simulink model "H8_pruebas_SIL"  (R2022b)
settings: Solver=VariableStepAuto  StartTime=0.0  StopTime=5  MaxStep=1e-3  RelTol=1e-3
InitFcn:
  | load("ems.mat");
  | load("hems.mat");
  | load('fuerzasY_LIM.mat')
  | load('matrices_linealizacion_6gdl.mat')
  | m = 200;
  | g = 9.81;
  | 
  | x_lev12 = 0.50086;
  | x_lev34 = 0.48414;
  | x_guid12 = 0.50503;
  | x_guid34 = 0.48831;
  | x_lim = 0.00778;
  | 
  | y_lev13 = 0.23523;
  | y_lev24 = 0.23827;
  | y_guid13 = 0.2372;
  | y_guid24 = 0.2402;
  | y_lim = 0.00154;
  | y_brk = 0.21552;
  | 
  | z_lev = 0.07138;
  | z_guid = 0.04113;
  | z_lim = 0.09146;
  | z_brk = 0.03941;
  | 
  | kp_lev = 50;
  | ki_lev = 400;
  | kp_guid = 6;
  | ki_guid = 46.5;
  | 
  | Imax_lev = 50;
  | Imin_lev = -50;
  | Imax_guid = 50;
  | Imin_guid = 0;
  | 
  | cg_nom=0.61448;
  | lev_nom=0.01965;
  | cg_suelo=0.61733;
  | cg_techo=0.60483;
  | 
  | I = [43.082 0 0; 0 26.887 -0; 0 0 29.297];
  | 
  | fs_current = 20000;
  | fl_current = 10000;
  | var_current = 0.052125100064495;
  | offset_current = 0.001065378087271;
  | 
  | fs_airgap = 20000;
  | fl_airgap = 7500;
  | var_airgap = 1.112140361208638e-08;
  | offset_airgap = 0;
  | airgap_min = 80/1000;
  | airgap_max = 115/1000;
  | 
  | current_filter_order = 20;
  | 
  | airgap_filter_order = 20;
  | N=16;
values from neighbouring files (symbols this model uses):
  A6 = [0 0 0 0 0 0 0 0 0 0 0 0 ... (100 elements, 10x10)]    [matrices_linealizacion_6gdl.mat]    (also in matrices_linealizacion_6gdl2.mat)
  B6 = [0 0 0 0 0 0 -0.0459993641186 -0.0505798680894 0.151580453785 0 0 0 ... (80 elements, 10x8)]    [matrices_linealizacion_6gdl.mat]    (also in matrices_linealizacion_6gdl2.mat)
  C6 = [1 0 0 0 0 0 0 0 0 0 0 1 ... (100 elements, 10x10)]    [matrices_linealizacion_6gdl.mat]    (also in matrices_linealizacion_6gdl2.mat)
  current = [0 10 20 30 40 50 60 70 80 90 100]    [fuerzasY_LIM.mat]
  D6 = [0 0 0 0 0 0 0 0 0 0 0 0 ... (80 elements, 10x8)]    [matrices_linealizacion_6gdl.mat]    (also in matrices_linealizacion_6gdl2.mat)
  FuerzaRail_Y = [0 0 0 0 0 0 0 0.015951701 0.168531476 0.364402347 0.577209778 0.832001165 ... (77 elements, 7x11)]    [fuerzasY_LIM.mat]
  hems =     [hems.mat]
  Ka = [0 0 0 0 4539.83149439 -4539.83149439 4539.83149439 -4539.83149439 -5130.48383819 -5130.48383819 -5130.48383819 -5130.48383819 ... (120 elements, 8x15)]    [Ka_reajustada.mat]    (also in matrices_linealizacion_6gdl.mat = [0 0 0 0 6002.75566687 -6002.75566687 6002.75566687 -6002.75; matrices_linealizacion_6gdl2.mat = [0 0 0 0 1200.55113337 -1200.55113337 1200.55113337 -1200.55)
  Y = [0 1 2 3 4 5 6]    [fuerzasY_LIM.mat]
undefined symbols (not defined in the file or in its folder): DiscIntNeverNeededParam, ems, magnitude
libraries: slpidlib x16, simulink x5
(part 1 of 2)
settings Model: Creator=USUARIO  LastModifiedBy=USUARIO
settings SolverCC: ZeroCrossAlgorithm=Adaptive
settings DebuggingCC: ModelReferenceExtraNoncontSigs=warning

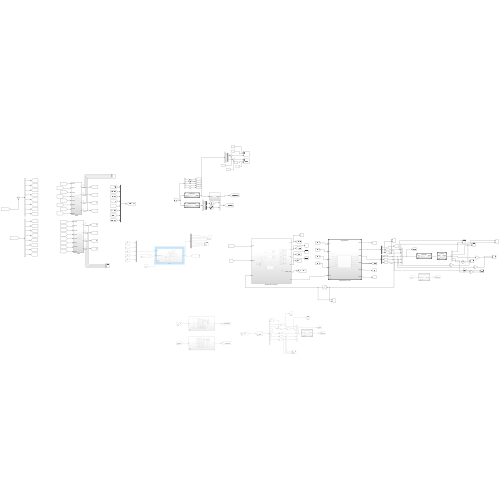
[thumbnail: Simulink's stored preview of the top-level diagram]
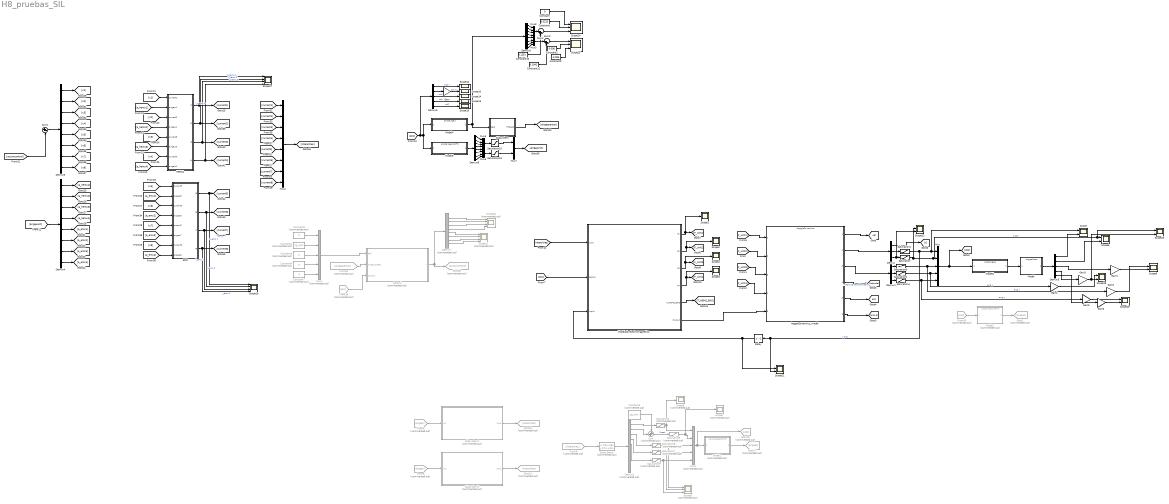
== system H8_pruebas_SIL ==
  Constant : Constant  Value=0
  Constant1 : Constant  Value=0.0225
  Constant10 : Constant  Value=0.1251
  Constant11 : Constant  Value=0.1042
  Constant2 : Constant  Value=0.006
  Constant3 : Constant  Commented=on  Value=cg_nom
  Constant4 : Constant  Commented=on  Value=cg_nom
  Constant{5..8} (4 alike) : Constant  Commented=on  Value=0
  Constant9 : Constant  Value=-0.006
  Control : Subsystem  Commented=on
  Delay : Delay  DelayLength=1  InitialCondition=0.001
  Demux : Demux  Outputs=3
  Demux1 : Demux  Outputs=3
  Demux2 : Demux  Commented=on  Outputs=10
      settings: DisplayOption=none
  Demux3 : Demux  Outputs=5
  Demux{4..5,8..9} (4 alike) : Demux  Outputs=8
  Demux6 : Demux  Outputs=5
  Demux7 : Demux  Commented=on  Outputs=8
  EMS : Subsystem
  From30 : From  Commented=on  GotoTag=airgapsensor
  From39 : From  Commented=on  GotoTag=pos
  From40 : From  Commented=on  GotoTag=pos
  From6 : From  Commented=on  GotoTag=airgaps
  From8 : From  Commented=on  GotoTag=airgaps
  From9 : From  Commented=on  GotoTag=Intensities
  Gain : Gain  Gain=1000
  Gain{1..6} (6 alike) : Gain  Gain=180/pi
  Goto1 : Goto  Commented=on  GotoTag=airgaps
  Goto13 : Goto  Commented=on  GotoTag=Intensities
  Goto16 : Goto  Commented=on  GotoTag=Intensities
  Goto17 : Goto  Commented=on  GotoTag=airgaps
  Goto18 : Goto  Commented=on  GotoTag=pos
  Goto38 : Goto  Commented=on  GotoTag=accioncontrol
  HEMS1 : Subsystem
  Model : ModelReference  ModelNameDialog=airgap2pos.slx  SimulationMode=Normal  ModelReferenceVersion=1.8
  Model1 : ModelReference  Commented=on  ModelNameDialog=pos2airgapUNITS.slx  SimulationMode=Normal  ModelReferenceVersion=1.5
  Model2 : ModelReference  Commented=on  ModelNameDialog=pos2airgapUNITS.slx  SimulationMode=Normal  ModelReferenceVersion=1.5
  Model4 : ModelReference  ModelNameDialog=pos2airgap.slx  SimulationMode=Normal  ModelReferenceVersion=1.7
  Model5 : ModelReference  ModelNameDialog=pos2airgapUNITS.slx  SimulationMode=Normal  ModelReferenceVersion=1.5
  Model6 : ModelReference  ModelNameDialog=pos2airgap.slx  SimulationMode=Normal  ModelReferenceVersion=1.7
  Modelado electromagnetico : Subsystem
  Mux : Mux  Inputs=5
  Mux1 : Mux  Commented=on  Inputs=5
  Mux2 : Mux  Inputs=8
  Mux{3,5..6,8} (4 alike) : Mux
  Mux4 : Mux  Commented=on  Inputs=5
  Mux7 : Mux  Inputs=2
  Saturation : Saturate  UpperLimit=cg_suelo  LowerLimit=cg_techo
  Saturation1 : Saturate  UpperLimit=0.012  LowerLimit=-0.012
  Saturation15 : Saturate  UpperLimit=0.0225  LowerLimit=0.01
  Saturation16 : Saturate  UpperLimit=0.024  LowerLimit=0
  Saturation2 : Saturate  UpperLimit=0.01268  LowerLimit=-0.01268
  Saturation3 : Saturate  UpperLimit=0.0476  LowerLimit=-0.0476
  Saturation4 : Saturate  UpperLimit=0.024  LowerLimit=-0.024
  Saturation5 : Saturate  Commented=on  UpperLimit=cg_suelo  LowerLimit=cg_techo
  Saturation6 : Saturate  Commented=on  UpperLimit=0.012  LowerLimit=-0.012
  Saturation7 : Saturate  Commented=on  UpperLimit=0.01268  LowerLimit=-0.01268
  Saturation8 : Saturate  Commented=on  UpperLimit=0.0476  LowerLimit=-0.0476
  Saturation9 : Saturate  Commented=on  UpperLimit=0.024  LowerLimit=-0.024
  Scope{,5..6,18..19,21..23} (8 alike) : Scope  NumInputPorts=2
  Scope{1..4,10,12..15} (9 alike) : Scope
  Scope11 : Scope  Commented=on  NumInputPorts=4
  Scope16 : Scope  NumInputPorts=4
  Scope24 : Scope  NumInputPorts=3
  Scope25 : Scope  NumInputPorts=3
  Scope26 : Scope  Commented=on  NumInputPorts=4
  Scope27 : Scope  NumInputPorts=4
  Scope7 : Scope  Commented=on
  Scope8 : Scope  Commented=on
  Scope9 : Scope  Commented=on  NumInputPorts=3
  State-Space : StateSpace  Commented=on  A=A6  B=B6  C=C6  D=D6  InitialCondition=[-0.001 0.001 0.001 -0.001 0.001 0 0 0 0 0]
  Subsystem : Subsystem
  Subsystem1 : Subsystem  Commented=on
  Subsystem2 : Subsystem  Commented=on
  Sum : Sum  Commented=on  Inputs=++|
  Sum1 : Sum  Inputs=|+-
  Sum2 : Sum  Inputs=|-+
  Sum3 : Sum  Inputs=|-+
  boggieDynamics_model : ModelReference  ModelNameDialog=boggieDynamics.mdl  SimulationMode=Normal  ModelReferenceVersion=1.43
  tag scope: acc=global, vel=global
  wires:
  [F_Unit4] -> boggieDynamics_model/4
  [F_Unit3] -> boggieDynamics_model/3
  [F_Unit2] -> boggieDynamics_model/2
  boggieDynamics_model/4 -> [Attitude]  "matriz de transformacion"
  [F_Unit1] -> boggieDynamics_model/1
  boggieDynamics_model/3 -> Demux1/1
  Mux/1 -> Model6/1, [pos]
  boggieDynamics_model/2 -> Demux/1
  Demux/3 -> Scope22/2, Saturation/1
  Demux/1 -> [x]
  boggieDynamics_model/1 -> [vel]
  Demux/2 -> Saturation1/1
  boggieDynamics_model/5 -> [acc]
  boggieDynamics_model/6 -> [angvel]
  [pos] -> Modelado electromagnetico/2(Ag_lev)
  [Intensities] -> Modelado electromagnetico/1(I_lev)
  Modelado electromagnetico/3(F3) -> Scope4/1, [F_Unit3]
  Modelado electromagnetico/2(F2) -> Scope2/1, [F_Unit2]
  Modelado electromagnetico/1(F1) -> Scope1/1, [F_Unit1]
  Modelado electromagnetico/5(T_HEMS_EMS) -> [T_HEMS_EMS]
  Demux1/1 -> Saturation3/1
  Demux1/2 -> Saturation2/1
  Demux1/3 -> Saturation4/1
  Model2/1 -> Goto1/1
  Saturation1/1 -> Scope21/2, Delay/1, Scope/1, Mux/1  "y pos"
  Saturation/1 -> Scope22/1, Scope23/1, Scope5/1, Mux/2  "z pos"
  Saturation3/1 -> Gain2/1, Mux/3  "ang x"
  Saturation2/1 -> Gain4/1, Mux/4  "ang y"
  Saturation4/1 -> Gain5/1, Mux/5  "ang z"
  Modelado electromagnetico/4(F4) -> Scope3/1, [F_Unit4]
  Subsystem1/1(Out1) -> Goto16/1
  From8/1 -> Subsystem1/1(In1)
  From6/1 -> Subsystem2/1(In1)
  Subsystem2/1(Out1) -> Goto13/1
  From9/1 -> State-Space/1
  State-Space/1 -> Demux2/1
  Demux2/3 -> Saturation8/1
  Saturation7/1 -> Scope9/2, Mux1/4
  Saturation8/1 -> Mux1/3, Scope9/1
  Demux2/4 -> Saturation7/1
  Saturation9/1 -> Mux1/5, Scope9/3
  Model1/1 -> Goto17/1
  Demux2/5 -> Saturation9/1
  Saturation6/1 -> Mux1/1, Scope8/1
  Demux2/1 -> Saturation6/1
  Mux1/1 -> Model1/1, Goto18/1
  Constant3/1 -> Sum/1
  Demux2/2 -> Sum/2
  Sum/1 -> Saturation5/1  "lineal"
  Saturation5/1 -> Mux1/2, Scope7/1
  Demux4/5 -> [a_ems1]
  [a_hems1] -> HEMS1/2(airgap1)
  Demux4/7 -> [a_ems3]
  [current8] -> Mux2/8
  Demux4/8 -> [a_ems4]
  Demux5/5 -> [c5]
  Demux4/6 -> [a_ems2]
  [accioncontrol] -> Sum1/2
  From30/1 -> Control/2(airgaps_Real)
  Demux4/2 -> [a_hems2]
  Demux5/2 -> [c2]
  Demux5/4 -> [c4]
  Mux7/1 -> [airgapunit]
  Saturation16/1 -> Mux7/2
  Saturation15/1 -> Mux7/1
  Demux7/8 -> Scope11/4
  Mux5/1 -> Saturation16/1
  Demux8/6 -> Mux5/2
  Demux8/7 -> Mux5/3
  Mux6/1 -> Saturation15/1
  Demux8/3 -> Mux6/3
  Demux8/5 -> Mux5/1
  Demux5/3 -> [c3]
  Demux8/2 -> Mux6/2
  Sum1/1 -> Demux5/1
  [current5] -> Mux2/5
  Demux6/3 -> Scope14/1  "rotX"
  [current6] -> Mux2/6
  [current7] -> Mux2/7
  Demux7/5 -> Scope11/1
  Constant5/1 -> Mux4/3
  [a_ems1] -> EMS/2(airgap5)
  Mux4/1 -> Control/1(Ref)
  Demux6/5 -> Scope15/1  "rotZ"
  Demux5/1 -> [c1]
  Demux7/6 -> Scope11/2
  Constant6/1 -> Mux4/4
  [current1] -> Mux2/1
  [a_hems3] -> HEMS1/6(airgap3)
  [a_ems3] -> EMS/6(airgap7)
  [a_hems4] -> HEMS1/8(airgap4)
  Demux4/1 -> [a_hems1]
  [a_ems4] -> EMS/8(airgap8)
  [a_hems2] -> HEMS1/4(airgap2)
  Demux5/7 -> [c7]
  [current3] -> Mux2/3
  Model4/1 -> Demux9/1, Subsystem/1(Real)
  Demux6/4 -> Scope13/1  "rotY"
  Demux7/7 -> Scope11/3
  Demux4/4 -> [a_hems4]
  Gain/1 -> Scope10/1  "pos Z"
  Constant4/1 -> Mux4/2
  Constant8/1 -> Mux4/1
  Demux5/6 -> [c6]
  Constant7/1 -> Mux4/5
  Demux4/3 -> [a_hems3]
  Demux8/8 -> Mux5/4
  Demux6/2 -> Gain/1
  Demux8/1 -> Mux6/1
  [current2] -> Mux2/2
  [a_ems2] -> EMS/4(airgap6)
  [current4] -> Mux2/4
  Demux5/8 -> [c8]
  Mux2/1 -> [Intensities]
  Demux6/1 -> Scope12/1  "pos Y"
  Demux8/4 -> Mux6/4
  [airgapunit] -> Demux4/1
  [pos] -> Demux6/1, Model4/1, Model5/1
  Model5/1 -> Demux8/1
  Control/1(I) -> Goto38/1, Demux7/1
  From39/1 -> Control/3(Output)
  From40/1 -> Model2/1
  Model6/1 -> Model/1
  Model/1 -> Demux3/1
  Demux3/1 -> Scope/2
  Demux3/2 -> Scope5/2
  Demux3/3 -> Gain1/1
  Demux3/4 -> Gain3/1
  Demux3/5 -> Gain6/1
  Modelado electromagnetico/6(Output) -> boggieDynamics_model/5
  Delay/1 -> Scope21/1, Modelado electromagnetico/3(Input)
  Gain1/1 -> Scope6/2
  Gain2/1 -> Scope6/1
  Gain3/1 -> Scope23/2, Scope18/2
  Gain4/1 -> Scope18/1
  Gain5/1 -> Scope19/1
  Gain6/1 -> Scope19/2
  Demux9/6 -> Mux3/2
  Demux9/8 -> Mux3/4
  Demux9/4 -> Mux8/4
  Demux9/7 -> Mux3/3
  Demux9/5 -> Mux3/1
  Demux9/3 -> Mux8/3
  Demux9/1 -> Mux8/1
  Mux3/1 -> Sum3/1
  Mux8/1 -> Sum2/1
  Demux9/2 -> Mux8/2
  Sum2/1 -> Scope24/3
  Constant1/1 -> Scope24/2
  Constant/1 -> Scope24/1
  Sum3/1 -> Scope25/1
  Constant9/1 -> Scope25/3
  Constant2/1 -> Scope25/2
  Constant10/1 -> Sum2/2
  Constant11/1 -> Sum3/2
  Demux7/1 -> Scope26/1
  Demux7/2 -> Scope26/2
  Demux7/3 -> Scope26/3
  Demux7/4 -> Scope26/4
  [c4] -> HEMS1/7(current4)
  [c3] -> HEMS1/5(current3)
  [c2] -> HEMS1/3(current2)
  [c1] -> HEMS1/1(current1)
  HEMS1/1(I1) -> Scope27/1, [current1]  "I_hems 1"
  HEMS1/2(I2) -> Scope27/2, [current2]  "I_hems 2"
  HEMS1/3(I3) -> Scope27/3, [current3]  "I_hems 3"
  HEMS1/4(I4) -> Scope27/4, [current4]  "I_hems 4"
  EMS/1(I5) -> Scope16/1, [current5]  "I_ems 1"
  EMS/2(I6) -> Scope16/2, [current6]  "I_ems 1"
  EMS/3(I7) -> Scope16/3, [current7]  "I_ems 1"
  EMS/4(I8) -> Scope16/4, [current8]  "I_ems 1"
  [c8] -> EMS/7(current8)
  [c7] -> EMS/5(current7)
  [c6] -> EMS/3(current6)
  [c5] -> EMS/1(current5)
  Subsystem/1(Filtered) -> [airgapsensor]

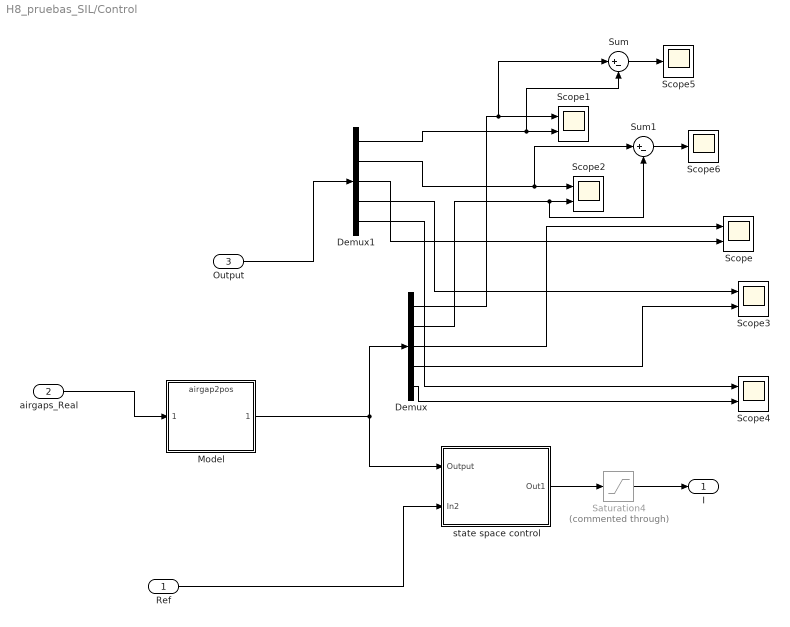
== system H8_pruebas_SIL/Control ==
  Ref : Inport
  airgaps_Real : Inport  Port=2
  Output : Inport  Port=3
  Demux : Demux  Outputs=5
  Demux1 : Demux  Outputs=5
  Model : ModelReference  ModelNameDialog=airgap2pos.slx  SimulationMode=Normal  ModelReferenceVersion=1.8
  Saturation4 : Saturate  Commented=through  UpperLimit=55  LowerLimit=-55
  Scope{,1..4} (5 alike) : Scope  NumInputPorts=2
  Scope5 : Scope
  Scope6 : Scope
  Sum : Sum  Inputs=|+-
  Sum1 : Sum  Inputs=|+-
  state space control : Subsystem
  I : Outport
  wires:
  airgaps_Real/1 -> Model/1
  Saturation4/1 -> I/1
  Model/1 -> state space control/1(Output), Demux/1
  Ref/1 -> state space control/2(In2)
  state space control/1(Out1) -> Saturation4/1
  Demux/1 -> Sum/1, Scope1/1
  Demux/3 -> Scope/1
  Demux/4 -> Scope3/2
  Demux/2 -> Scope2/2, Sum1/2
  Demux1/1 -> Sum/2, Scope1/2
  Demux1/2 -> Sum1/1, Scope2/1
  Demux1/3 -> Scope/2
  Demux1/4 -> Scope3/1
  Demux1/5 -> Scope4/1
  Demux/5 -> Scope4/2
  Sum/1 -> Scope5/1
  Sum1/1 -> Scope6/1
  Output/1 -> Demux1/1

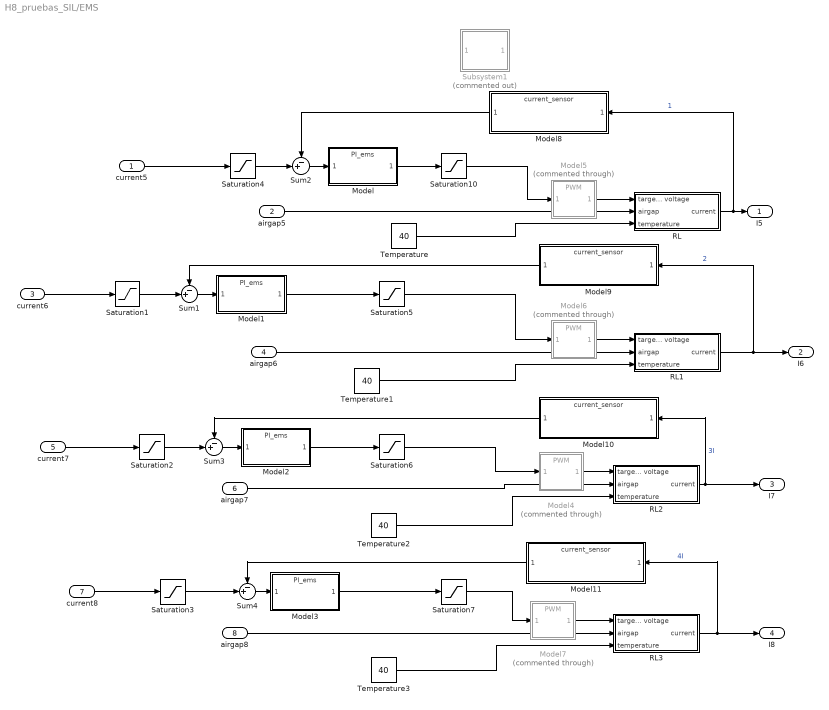
== system H8_pruebas_SIL/EMS ==
  current5 : Inport
  airgap5 : Inport  Port=2
  current6 : Inport  Port=3
  airgap6 : Inport  Port=4
  current7 : Inport  Port=5
  airgap7 : Inport  Port=6
  current8 : Inport  Port=7
  airgap8 : Inport  Port=8
  Model{,1..3} (4 alike) : ModelReference  ModelNameDialog=PI_ems.slx  SimulationMode=Normal  ModelReferenceVersion=1.3
  Model{8..11} (4 alike) : ModelReference  ModelNameDialog=current_sensor.slx  SimulationMode=Normal  ModelReferenceVersion=1.2
  Model{4..7} (4 alike) : ModelReference  Commented=through  ModelNameDialog=PWM.slx  SimulationMode=Normal  ModelReferenceVersion=1.7
  RL : Subsystem
  RL1 : Subsystem
  RL2 : Subsystem
  RL3 : Subsystem
  Saturation{1..4} (4 alike) : Saturate  UpperLimit=50  LowerLimit=0
  Saturation{5..7,10} (4 alike) : Saturate  UpperLimit=200  LowerLimit=-200
  Subsystem1 : Subsystem  Commented=on
  Sum{1..4} (4 alike) : Sum  Inputs=-+|
  Temperature{,1..3} (4 alike) : Constant  Value=40
  I5 : Outport
  I6 : Outport  Port=2
  I7 : Outport  Port=3
  I8 : Outport  Port=4
  wires:
  Temperature/1 -> RL/3(temperature)
  airgap5/1 -> RL/2(airgap)
  Temperature3/1 -> RL3/3(temperature)
  RL/1(current) -> I5/1, Model8/1  "1"
  Temperature1/1 -> RL1/3(temperature)
  Temperature2/1 -> RL2/3(temperature)
  RL3/1(current) -> I8/1, Model11/1  "4I"
  airgap6/1 -> RL1/2(airgap)
  RL1/1(current) -> I6/1, Model9/1  "2"
  RL2/1(current) -> I7/1, Model10/1  "3I"
  airgap7/1 -> RL2/2(airgap)
  airgap8/1 -> RL3/2(airgap)
  Sum2/1 -> Model/1
  Sum1/1 -> Model1/1
  Sum3/1 -> Model2/1
  Sum4/1 -> Model3/1
  Model/1 -> Saturation10/1
  Model3/1 -> Saturation7/1
  Model2/1 -> Saturation6/1
  Model1/1 -> Saturation5/1
  Saturation4/1 -> Sum2/2
  Saturation1/1 -> Sum1/2
  Saturation2/1 -> Sum3/2
  Saturation3/1 -> Sum4/2
  current5/1 -> Saturation4/1
  current6/1 -> Saturation1/1
  current7/1 -> Saturation2/1
  current8/1 -> Saturation3/1
  Saturation7/1 -> Model7/1
  Saturation6/1 -> Model4/1
  Saturation5/1 -> Model6/1
  Saturation10/1 -> Model5/1
  Model6/1 -> RL1/1(target voltage)
  Model4/1 -> RL2/1(target voltage)
  Model5/1 -> RL/1(target voltage)
  Model7/1 -> RL3/1(target voltage)
  Model8/1 -> Sum2/1
  Model9/1 -> Sum1/1
  Model10/1 -> Sum3/1
  Model11/1 -> Sum4/1

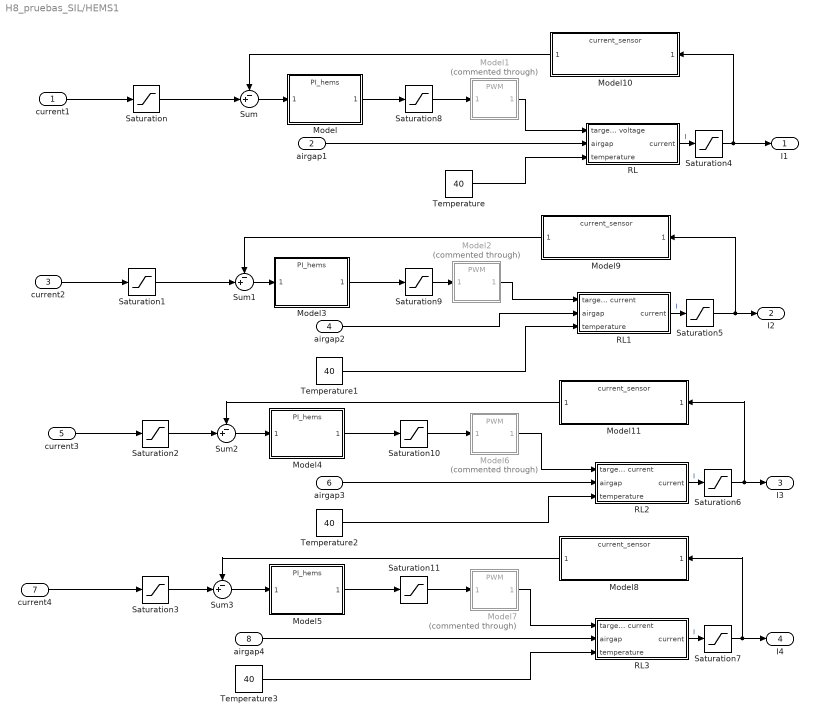
== system H8_pruebas_SIL/HEMS1 ==
  current1 : Inport
  airgap1 : Inport  Port=2
  current2 : Inport  Port=3
  airgap2 : Inport  Port=4
  current3 : Inport  Port=5
  airgap3 : Inport  Port=6
  current4 : Inport  Port=7
  airgap4 : Inport  Port=8
  Model{,3..5} (4 alike) : ModelReference  ModelNameDialog=PI_hems.slx  SimulationMode=Normal  ModelReferenceVersion=1.5
  Model{1..2,6..7} (4 alike) : ModelReference  Commented=through  ModelNameDialog=PWM.slx  SimulationMode=Normal  ModelReferenceVersion=1.7
  Model{8..11} (4 alike) : ModelReference  ModelNameDialog=current_sensor.slx  SimulationMode=Normal  ModelReferenceVersion=1.2
  RL : Subsystem
  RL1 : Subsystem
  RL2 : Subsystem
  RL3 : Subsystem
  Saturation{,1..7} (8 alike) : Saturate  UpperLimit=50  LowerLimit=-50
  Saturation{8..11} (4 alike) : Saturate  UpperLimit=200  LowerLimit=-200
  Sum{,1..3} (4 alike) : Sum  Inputs=-+|
  Temperature{,1..3} (4 alike) : Constant  Value=40
  I1 : Outport
  I2 : Outport  Port=2
  I3 : Outport  Port=3
  I4 : Outport  Port=4
  wires:
  Temperature/1 -> RL/3(temperature)
  Model3/1 -> Saturation9/1
  Model5/1 -> Saturation11/1
  Model/1 -> Saturation8/1
  airgap1/1 -> RL/2(airgap)
  Temperature3/1 -> RL3/3(temperature)
  RL/1(current) -> Saturation4/1  "I"
  Temperature1/1 -> RL1/3(temperature)
  Temperature2/1 -> RL2/3(temperature)
  Model4/1 -> Saturation10/1
  RL3/1(current) -> Saturation7/1  "I"
  airgap2/1 -> RL1/2(airgap)
  RL1/1(current) -> Saturation5/1  "I"
  RL2/1(current) -> Saturation6/1  "I"
  airgap3/1 -> RL2/2(airgap)
  airgap4/1 -> RL3/2(airgap)
  Sum/1 -> Model/1
  Sum1/1 -> Model3/1
  Sum2/1 -> Model4/1
  Sum3/1 -> Model5/1
  Saturation2/1 -> Sum2/2
  Saturation1/1 -> Sum1/2
  Saturation/1 -> Sum/2
  Saturation3/1 -> Sum3/2
  current1/1 -> Saturation/1
  current4/1 -> Saturation3/1
  current3/1 -> Saturation2/1
  current2/1 -> Saturation1/1
  Saturation4/1 -> I1/1, Model10/1
  Saturation5/1 -> I2/1, Model9/1
  Saturation7/1 -> I4/1, Model8/1
  Saturation6/1 -> I3/1, Model11/1
  Saturation8/1 -> Model1/1
  Saturation9/1 -> Model2/1
  Saturation10/1 -> Model6/1
  Saturation11/1 -> Model7/1
  Model1/1 -> RL/1(target voltage)
  Model2/1 -> RL1/1(target current)
  Model6/1 -> RL2/1(target current)
  Model7/1 -> RL3/1(target current)
  Model8/1 -> Sum3/1
  Model9/1 -> Sum1/1
  Model10/1 -> Sum/1
  Model11/1 -> Sum2/1

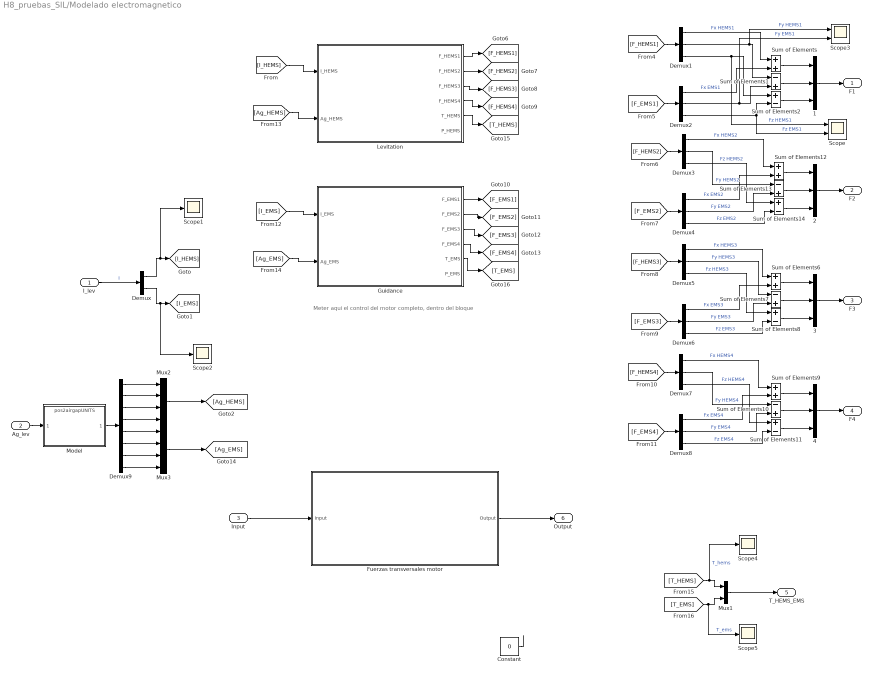
== system H8_pruebas_SIL/Modelado electromagnetico ==
  note: Meter aqui el control del motor completo, dentro del bloque
  I_lev : Inport
  Ag_lev : Inport  Port=2
  Input : Inport  Port=3
  {1..4} (4 alike) : Mux  Inputs=3
  Constant : Constant  Value=0
  Demux : Demux  Outputs=2
  Demux{1..8} (8 alike) : Demux  Outputs=3
  Demux9 : Demux  Outputs=8
  Fuerzas transversales motor : Subsystem
  Guidance : Subsystem
  Levitation : Subsystem
  Model : ModelReference  ModelNameDialog=pos2airgapUNITS.slx  SimulationMode=Normal  ModelReferenceVersion=1.5
  Mux1 : Mux  Inputs=2
  Mux2 : Mux
  Mux3 : Mux
  Scope : Scope  NumInputPorts=2
  Scope{1..2,4..5} (4 alike) : Scope
  Scope3 : Scope  NumInputPorts=2
  Sum of Elements{,6,9,12} (4 alike) : Sum
  Sum of Elements{1,7,10,13} (4 alike) : Sum  Inputs=-+
  Sum of Elements{2,8,11,14} (4 alike) : Sum  Inputs=+-
  F1 : Outport
  F2 : Outport  Port=2
  F3 : Outport  Port=3
  F4 : Outport  Port=4
  T_HEMS_EMS : Outport  Port=5
  Output : Outport  Port=6
  wires:
  I_lev/1 -> Demux/1  "I"
  Demux/1 -> Scope1/1, [I_HEMS]
  Demux/2 -> Scope2/1, [I_EMS]
  [I_HEMS] -> Levitation/1(I_HEMS)
  Levitation/1(F_HEMS1) -> [F_HEMS1]
  Levitation/2(F_HEMS2) -> [F_HEMS2]
  Levitation/3(F_HEMS3) -> [F_HEMS3]
  Levitation/4(F_HEMS4) -> [F_HEMS4]
  Sum of Elements/1 -> 1/1
  1/1 -> F1/1
  Sum of Elements1/1 -> 1/2
  Sum of Elements2/1 -> 1/3
  2/1 -> F2/1
  [F_HEMS1] -> Demux1/1
  Demux1/1 -> Sum of Elements/1  "Fx HEMS1"
  Demux1/2 -> Scope3/1, Sum of Elements1/1  "Fy HEMS1"
  Demux1/3 -> Scope/1, Sum of Elements2/1  "Fz HEMS1"
  3/1 -> F3/1
  Sum of Elements8/1 -> 3/3
  Sum of Elements6/1 -> 3/1
  Sum of Elements7/1 -> 3/2
  4/1 -> F4/1
  Sum of Elements11/1 -> 4/3
  Sum of Elements9/1 -> 4/1
  Sum of Elements10/1 -> 4/2
  Guidance/2(F_EMS2) -> [F_EMS2]
  Guidance/3(F_EMS3) -> [F_EMS3]
  Guidance/4(F_EMS4) -> [F_EMS4]
  Guidance/1(F_EMS1) -> [F_EMS1]
  Demux2/1 -> Sum of Elements/2  "Fx EMS1"
  [F_EMS1] -> Demux2/1
  Demux2/2 -> Scope3/2, Sum of Elements1/2  "Fy EMS1"
  Demux2/3 -> Sum of Elements2/2, Scope/2  "Fz EMS1"
  [F_EMS2] -> Demux4/1
  Demux4/1 -> Sum of Elements12/2  "Fx EMS2"
  Demux4/2 -> Sum of Elements13/2  "Fy EMS2"
  Sum of Elements14/1 -> 2/3
  Demux3/1 -> Sum of Elements12/1  "Fx HEMS2"
  [F_HEMS2] -> Demux3/1
  Demux3/2 -> Sum of Elements13/1  "Fy HEMS2"
  Demux3/3 -> Sum of Elements14/1  "Fz HEMS2"
  Sum of Elements13/1 -> 2/2
  Sum of Elements12/1 -> 2/1
  Demux4/3 -> Sum of Elements14/2  "Fz EMS2"
  Demux5/3 -> Sum of Elements8/1  "Fz HEMS3"
  Demux5/2 -> Sum of Elements7/1  "Fy HEMS3"
  [F_HEMS3] -> Demux5/1
  Demux6/3 -> Sum of Elements8/2  "Fz EMS3"
  [F_EMS3] -> Demux6/1
  Demux6/1 -> Sum of Elements6/2  "Fx EMS3"
  Demux5/1 -> Sum of Elements6/1  "Fx HEMS3"
  Demux6/2 -> Sum of Elements7/2  "Fy EMS3"
  Demux7/3 -> Sum of Elements11/1  "Fz HEMS4"
  Demux8/3 -> Sum of Elements11/2  "Fz EMS4"
  Demux8/2 -> Sum of Elements10/2  "Fy EMS4"
  Demux7/2 -> Sum of Elements10/1  "Fy HEMS4"
  Demux7/1 -> Sum of Elements9/1  "Fx HEMS4"
  Demux8/1 -> Sum of Elements9/2  "Fx EMS4"
  [F_HEMS4] -> Demux7/1
  [F_EMS4] -> Demux8/1
  [I_EMS] -> Guidance/1(I_EMS)
  Ag_lev/1 -> Model/1
  [Ag_HEMS] -> Levitation/2(Ag_HEMS)
  [Ag_EMS] -> Guidance/2(Ag_EMS)
  Levitation/5(T_HEMS) -> [T_HEMS]
  Guidance/5(T_EMS) -> [T_EMS]
  Mux1/1 -> T_HEMS_EMS/1
  [T_HEMS] -> Scope4/1, Mux1/1  "T_hems"
  [T_EMS] -> Scope5/1, Mux1/2  "T_ems"
  Model/1 -> Demux9/1
  Demux9/1 -> Mux2/1
  Demux9/2 -> Mux2/2
  Demux9/3 -> Mux2/3
  Demux9/4 -> Mux2/4
  Mux2/1 -> [Ag_HEMS]
  Demux9/5 -> Mux3/1
  Demux9/7 -> Mux3/3
  Mux3/1 -> [Ag_EMS]
  Demux9/6 -> Mux3/2
  Demux9/8 -> Mux3/4
  Input/1 -> Fuerzas transversales motor/1(Input)
  Fuerzas transversales motor/1(Output) -> Output/1
  Constant/1 -> ?

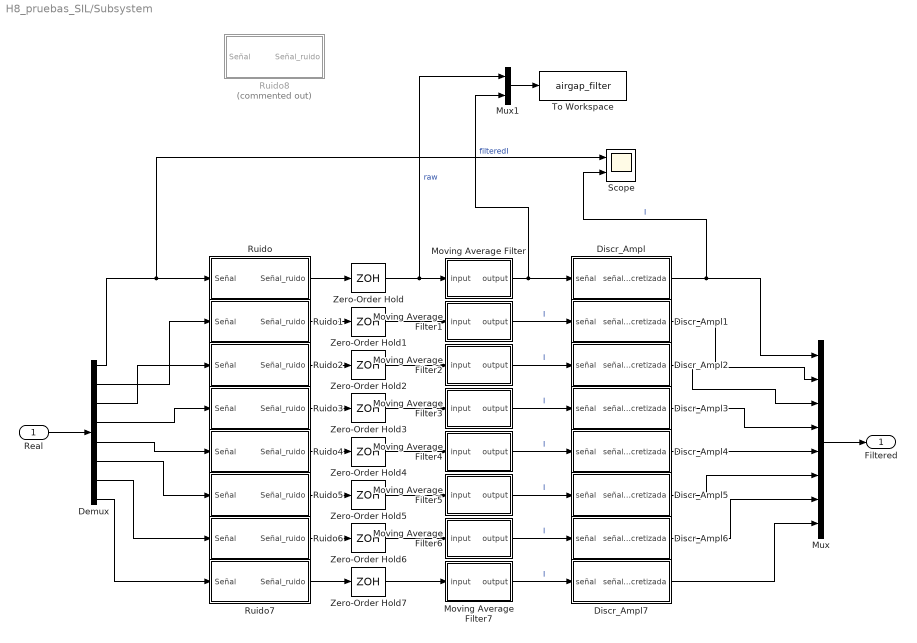
== system H8_pruebas_SIL/Subsystem ==
  Real : Inport
  Demux : Demux  Outputs=8
  Discr_Ampl : Subsystem  mask{N=(2^N)-1, Min=0.045, Max=0.125}
      mask prompts: N "Valores distintos (N)"; Min "Valor mínimo"; Max "Valor máximo"
      mask DialogControl DescGroupVar Prompt: Discretizacion_Amplitud
      mask DialogControl DescTextVar Prompt: Discretización en amplitud
  Discr_Ampl1 : Subsystem  mask{N=(2^N)-1, Min=0.045, Max=0.125}
      mask prompts: N "Valores distintos (N)"; Min "Valor mínimo"; Max "Valor máximo"
      mask DialogControl DescGroupVar Prompt: Discretizacion_Amplitud
      mask DialogControl DescTextVar Prompt: Discretización en amplitud
  Discr_Ampl2 : Subsystem  mask{N=(2^N)-1, Min=0.045, Max=0.125}
      mask prompts: N "Valores distintos (N)"; Min "Valor mínimo"; Max "Valor máximo"
      mask DialogControl DescGroupVar Prompt: Discretizacion_Amplitud
      mask DialogControl DescTextVar Prompt: Discretización en amplitud
  Discr_Ampl3 : Subsystem  mask{N=(2^N)-1, Min=0.045, Max=0.125}
      mask prompts: N "Valores distintos (N)"; Min "Valor mínimo"; Max "Valor máximo"
      mask DialogControl DescGroupVar Prompt: Discretizacion_Amplitud
      mask DialogControl DescTextVar Prompt: Discretización en amplitud
  Discr_Ampl4 : Subsystem  mask{N=(2^N)-1, Min=0.045, Max=0.125}
      mask prompts: N "Valores distintos (N)"; Min "Valor mínimo"; Max "Valor máximo"
      mask DialogControl DescGroupVar Prompt: Discretizacion_Amplitud
      mask DialogControl DescTextVar Prompt: Discretización en amplitud
  Discr_Ampl5 : Subsystem  mask{N=(2^N)-1, Min=0.045, Max=0.125}
      mask prompts: N "Valores distintos (N)"; Min "Valor mínimo"; Max "Valor máximo"
      mask DialogControl DescGroupVar Prompt: Discretizacion_Amplitud
      mask DialogControl DescTextVar Prompt: Discretización en amplitud
  Discr_Ampl6 : Subsystem  mask{N=(2^N)-1, Min=0.045, Max=0.125}
      mask prompts: N "Valores distintos (N)"; Min "Valor mínimo"; Max "Valor máximo"
      mask DialogControl DescGroupVar Prompt: Discretizacion_Amplitud
      mask DialogControl DescTextVar Prompt: Discretización en amplitud
  Discr_Ampl7 : Subsystem  mask{N=(2^N)-1, Min=0.045, Max=0.125}
      mask prompts: N "Valores distintos (N)"; Min "Valor mínimo"; Max "Valor máximo"
      mask DialogControl DescGroupVar Prompt: Discretizacion_Amplitud
      mask DialogControl DescTextVar Prompt: Discretización en amplitud
  Moving Average Filter : Subsystem  mask{M=airgap_filter_order, fs=-1}
      mask prompts: M "Orden del filtro (M)"; fs "Frecuencia de muestreo (fs)"
  Moving Average Filter1 : Subsystem  mask{M=airgap_filter_order, fs=-1}
      mask prompts: M "Orden del filtro (M)"; fs "Frecuencia de muestreo (fs)"
  Moving Average Filter2 : Subsystem  mask{M=airgap_filter_order, fs=-1}
      mask prompts: M "Orden del filtro (M)"; fs "Frecuencia de muestreo (fs)"
  Moving Average Filter3 : Subsystem  mask{M=airgap_filter_order, fs=-1}
      mask prompts: M "Orden del filtro (M)"; fs "Frecuencia de muestreo (fs)"
  Moving Average Filter4 : Subsystem  mask{M=airgap_filter_order, fs=-1}
      mask prompts: M "Orden del filtro (M)"; fs "Frecuencia de muestreo (fs)"
  Moving Average Filter5 : Subsystem  mask{M=airgap_filter_order, fs=-1}
      mask prompts: M "Orden del filtro (M)"; fs "Frecuencia de muestreo (fs)"
  Moving Average Filter6 : Subsystem  mask{M=airgap_filter_order, fs=-1}
      mask prompts: M "Orden del filtro (M)"; fs "Frecuencia de muestreo (fs)"
  Moving Average Filter7 : Subsystem  mask{M=airgap_filter_order, fs=-1}
      mask prompts: M "Orden del filtro (M)"; fs "Frecuencia de muestreo (fs)"
  Mux : Mux  Inputs=8
  Mux1 : Mux  Inputs=2
  Ruido : Subsystem  mask{M=0, V=var_airgap, T=1/fs_airgap}
      mask prompts: M "Media"; V "Varianza"; T "Periodo"
      mask DialogControl Ruido Prompt: Ruido
      mask DialogControl DescTextVar Prompt: Añade ruido gaussiano
  Ruido1 : Subsystem  mask{M=0, V=var_airgap, T=1/fs_airgap}
      mask prompts: M "Media"; V "Varianza"; T "Periodo"
      mask DialogControl Ruido Prompt: Ruido
      mask DialogControl DescTextVar Prompt: Añade ruido gaussiano
  Ruido2 : Subsystem  mask{M=0, V=var_airgap, T=1/fs_airgap}
      mask prompts: M "Media"; V "Varianza"; T "Periodo"
      mask DialogControl Ruido Prompt: Ruido
      mask DialogControl DescTextVar Prompt: Añade ruido gaussiano
  Ruido3 : Subsystem  mask{M=0, V=var_airgap, T=1/fs_airgap}
      mask prompts: M "Media"; V "Varianza"; T "Periodo"
      mask DialogControl Ruido Prompt: Ruido
      mask DialogControl DescTextVar Prompt: Añade ruido gaussiano
  Ruido4 : Subsystem  mask{M=0, V=var_airgap, T=1/fs_airgap}
      mask prompts: M "Media"; V "Varianza"; T "Periodo"
      mask DialogControl Ruido Prompt: Ruido
      mask DialogControl DescTextVar Prompt: Añade ruido gaussiano
  Ruido5 : Subsystem  mask{M=0, V=var_airgap, T=1/fs_airgap}
      mask prompts: M "Media"; V "Varianza"; T "Periodo"
      mask DialogControl Ruido Prompt: Ruido
      mask DialogControl DescTextVar Prompt: Añade ruido gaussiano
  Ruido6 : Subsystem  mask{M=0, V=var_airgap, T=1/fs_airgap}
      mask prompts: M "Media"; V "Varianza"; T "Periodo"
      mask DialogControl Ruido Prompt: Ruido
      mask DialogControl DescTextVar Prompt: Añade ruido gaussiano
  Ruido7 : Subsystem  mask{M=0, V=var_airgap, T=1/fs_airgap}
      mask prompts: M "Media"; V "Varianza"; T "Periodo"
      mask DialogControl Ruido Prompt: Ruido
      mask DialogControl DescTextVar Prompt: Añade ruido gaussiano
  Ruido8 : Subsystem  Commented=on  mask{M=0, V=5e-8, T=0.00001}
      mask prompts: M "Media"; V "Varianza"; T "Periodo"
      mask DialogControl Ruido Prompt: Ruido
      mask DialogControl DescTextVar Prompt: Añade ruido gaussiano
  Scope : Scope  NumInputPorts=2
  To Workspace : ToWorkspace  VariableName=airgap_filter  SaveFormat=Timeseries  SampleTime=-1
  Zero-Order Hold{,1..7} (8 alike) : ZeroOrderHold  SampleTime=1/fl_airgap
  Filtered : Outport
  wires:
  Real/1 -> Demux/1
  Demux/2 -> Ruido1/1(Señal)
  Demux/3 -> Ruido2/1(Señal)
  Demux/4 -> Ruido3/1(Señal)
  Demux/5 -> Ruido4/1(Señal)
  Demux/6 -> Ruido5/1(Señal)
  Demux/7 -> Ruido6/1(Señal)
  Demux/8 -> Ruido7/1(Señal)
  Mux/1 -> Filtered/1
  Discr_Ampl1/1(señal_discretizada) -> Mux/2
  Discr_Ampl2/1(señal_discretizada) -> Mux/3
  Discr_Ampl3/1(señal_discretizada) -> Mux/4
  Discr_Ampl4/1(señal_discretizada) -> Mux/5
  Discr_Ampl5/1(señal_discretizada) -> Mux/6
  Discr_Ampl6/1(señal_discretizada) -> Mux/7
  Discr_Ampl7/1(señal_discretizada) -> Mux/8
  Discr_Ampl/1(señal_discretizada) -> Scope/2, Mux/1  "I"
  Zero-Order Hold/1 -> Mux1/1, Moving Average Filter/1(input)  "raw"
  Ruido/1(Señal_ruido) -> Zero-Order Hold/1
  Moving Average Filter/1(output) -> Mux1/2, Discr_Ampl/1(señal)  "filteredI"
  Ruido1/1(Señal_ruido) -> Zero-Order Hold1/1
  Zero-Order Hold1/1 -> Moving Average Filter1/1(input)
  Moving Average Filter1/1(output) -> Discr_Ampl1/1(señal)  "I"
  Ruido2/1(Señal_ruido) -> Zero-Order Hold2/1
  Zero-Order Hold2/1 -> Moving Average Filter2/1(input)
  Moving Average Filter2/1(output) -> Discr_Ampl2/1(señal)  "I"
  Ruido3/1(Señal_ruido) -> Zero-Order Hold3/1
  Zero-Order Hold3/1 -> Moving Average Filter3/1(input)
  Moving Average Filter3/1(output) -> Discr_Ampl3/1(señal)  "I"
  Ruido4/1(Señal_ruido) -> Zero-Order Hold4/1
  Zero-Order Hold4/1 -> Moving Average Filter4/1(input)
  Moving Average Filter4/1(output) -> Discr_Ampl4/1(señal)  "I"
  Ruido5/1(Señal_ruido) -> Zero-Order Hold5/1
  Zero-Order Hold5/1 -> Moving Average Filter5/1(input)
  Moving Average Filter5/1(output) -> Discr_Ampl5/1(señal)  "I"
  Ruido6/1(Señal_ruido) -> Zero-Order Hold6/1
  Zero-Order Hold6/1 -> Moving Average Filter6/1(input)
  Moving Average Filter6/1(output) -> Discr_Ampl6/1(señal)  "I"
  Ruido7/1(Señal_ruido) -> Zero-Order Hold7/1
  Zero-Order Hold7/1 -> Moving Average Filter7/1(input)
  Moving Average Filter7/1(output) -> Discr_Ampl7/1(señal)  "I"
  Demux/1 -> Ruido/1(Señal), Scope/1
  Mux1/1 -> To Workspace/1

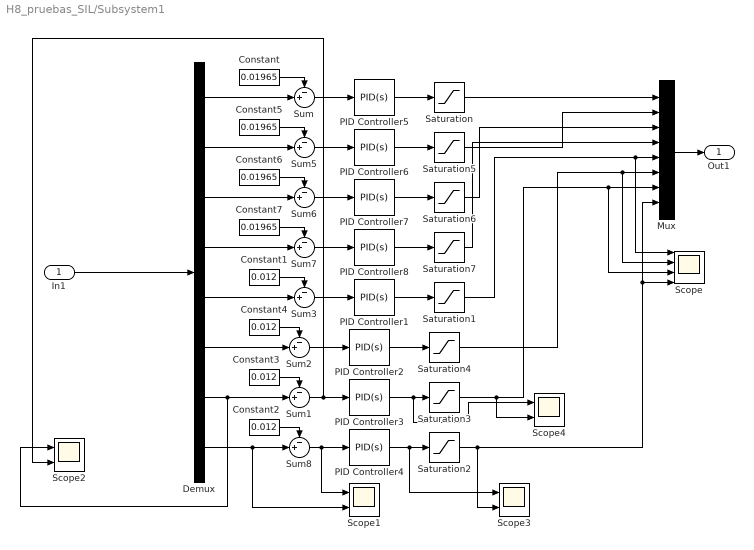
== system H8_pruebas_SIL/Subsystem1 ==
  In1 : Inport
  Constant{,5..7} (4 alike) : Constant  Value=0.01965
  Constant{1..4} (4 alike) : Constant  Value=0.012
  Demux : Demux  Outputs=8
  Mux : Mux  Inputs=8
  PID Controller{1..4} (4 alike) : slpidlib/PID Controller  Controller=PID  Form=Parallel  TimeDomain=Continuous-time  UseExternalTs=off  SampleTime=-1  IntegratorMethod=Forward Euler  FilterMethod=Forward Euler  ControllerParametersSource=internal  P=6490  I=15500  UseKiTs=off  D=100  N=1900  UseFilter=on  TunerSelectOption=Transfer Function Based (PID Tuner App)  InitialConditionSource=internal  InitialConditionForIntegrator=suelo  InitialConditionForFilter=0  DifferentiatorICPrevScaledInput=0  ExternalReset=none  TrackingMode=off  Kt=1  LimitOutput=off  SatLimitsSource=internal  UpperSaturationLimit=inf  LowerSaturationLimit=-inf  LinearizeAsGain=on  AntiWindupMode=none  Kb=1  LimitIntegrator=off  UpperIntegratorSaturationLimit=inf  LowerIntegratorSaturationLimit=-inf  POutMin=[]  POutMax=[]  IOutMin=[]  IOutMax=[]  DOutMin=[]  DOutMax=[]  NOutMin=[]  NOutMax=[]  SumOutMin=[]  SumOutMax=[]  SaturationOutMin=[]  SaturationOutMax=[]  PParamMin=[]  PParamMax=[]  IParamMin=[]  IParamMax=[]  DParamMin=[]  DParamMax=[]  NParamMin=[]  NParamMax=[]  KbParamMin=[]  KbParamMax=[]  KtParamMin=[]  KtParamMax=[]  KbOutMin=[]  KbOutMax=[]  KtOutMin=[]  KtOutMax=[]  IntegratorOutMin=[]  IntegratorOutMax=[]  FilterOutMin=[]  FilterOutMax=[]  SumI1OutMin=[]  SumI1OutMax=[]  SumI2OutMin=[]  SumI2OutMax=[]  SumI3OutMin=[]  SumI3OutMax=[]  SumI4OutMin=[]  SumI4OutMax=[]  SumDOutMin=[]  SumDOutMax=[]  DifferentiatorOutMin=[]  DifferentiatorOutMax=[]  FilterDiffOutCoefMin=[]  FilterDiffOutCoefMax=[]  ReciprocalOutMin=[]  ReciprocalOutMax=[]  SumDenOutMin=[]  SumDenOutMax=[]  SumNumOutMin=[]  SumNumOutMax=[]  DivideOutMin=[]  DivideOutMax=[]  UdiffTsProdOutMin=[]  UdiffTsProdOutMax=[]  NTsProdOutMin=[]  NTsProdOutMax=[]  UintegralTsProdOutMin=[]  UintegralTsProdOutMax=[]  UngainTsProdOutMin=[]  UngainTsProdOutMax=[]  ClampingZeroOutDataTypeStr=Inherit: Inherit via back propagation  ClampingZeroOutMin=[]  ClampingZeroOutMax=[]  FilterDenConstantOutDataTypeStr=Inherit: Inherit via back propagation  FilterDenConstantOutMin=[]  FilterDenConstantOutMax=[]  PCopyOutDataTypeStr=Inherit: Inherit via back propagation  PCopyOutMin=[]  PCopyOutMax=[]  NCopyOutDataTypeStr=Inherit: Inherit via back propagation  NCopyOutMin=[]  NCopyOutMax=[]  IntegratorContinuousStateAttributes=''  IntegratorStateMustResolveToSignalObject=off  IntegratorRTWStateStorageClass=Auto  FilterContinuousStateAttributes=''  FilterStateMustResolveToSignalObject=off  FilterRTWStateStorageClass=Auto  ParallelPVariant=InternalParameters  IdealPVariant=Disabled  IVariant=InternalParameters  DVariant=InternalParameters  IntegratorVariant=Continuous  SatVariant=Disabled  AWVariant=Passthrough  PCopyVariant=Disabled  TRVariant=Disabled  FdbkBlocksVariant=Forward  IdealPFdbkVariant=Disabled  SatFdbkVariant=Disabled  DerivativeFilterVariant=ContFilter  NVariant=InternalParameters  NCopyVariant=Disabled  FilterICVariant=InternalICsFilter  IntegratorICVariant=InternalICs  ExternalResetVariant=Disabled  TRSumVariant=Passthrough  SumFdbkVariant=Disabled  SumVariant=Sum_PID  TsampFilterVariant=InternalTs  TsampNgainVariant=Passthrough  TsampIntegralVariant=Passthrough  ExternalSaturationOutDataTypeStr=Inherit: Same as second input
  PID Controller{5..8} (4 alike) : slpidlib/PID Controller  Controller=PID  Form=Parallel  TimeDomain=Continuous-time  UseExternalTs=off  SampleTime=-1  IntegratorMethod=Forward Euler  FilterMethod=Forward Euler  ControllerParametersSource=internal  P=64900  I=155000  UseKiTs=off  D=1000  N=1900  UseFilter=on  TunerSelectOption=Transfer Function Based (PID Tuner App)  InitialConditionSource=internal  InitialConditionForIntegrator=suelo  InitialConditionForFilter=0  DifferentiatorICPrevScaledInput=0  ExternalReset=none  TrackingMode=off  Kt=1  LimitOutput=off  SatLimitsSource=internal  UpperSaturationLimit=inf  LowerSaturationLimit=-inf  LinearizeAsGain=on  AntiWindupMode=none  Kb=1  LimitIntegrator=off  UpperIntegratorSaturationLimit=inf  LowerIntegratorSaturationLimit=-inf  POutMin=[]  POutMax=[]  IOutMin=[]  IOutMax=[]  DOutMin=[]  DOutMax=[]  NOutMin=[]  NOutMax=[]  SumOutMin=[]  SumOutMax=[]  SaturationOutMin=[]  SaturationOutMax=[]  PParamMin=[]  PParamMax=[]  IParamMin=[]  IParamMax=[]  DParamMin=[]  DParamMax=[]  NParamMin=[]  NParamMax=[]  KbParamMin=[]  KbParamMax=[]  KtParamMin=[]  KtParamMax=[]  KbOutMin=[]  KbOutMax=[]  KtOutMin=[]  KtOutMax=[]  IntegratorOutMin=[]  IntegratorOutMax=[]  FilterOutMin=[]  FilterOutMax=[]  SumI1OutMin=[]  SumI1OutMax=[]  SumI2OutMin=[]  SumI2OutMax=[]  SumI3OutMin=[]  SumI3OutMax=[]  SumI4OutMin=[]  SumI4OutMax=[]  SumDOutMin=[]  SumDOutMax=[]  DifferentiatorOutMin=[]  DifferentiatorOutMax=[]  FilterDiffOutCoefMin=[]  FilterDiffOutCoefMax=[]  ReciprocalOutMin=[]  ReciprocalOutMax=[]  SumDenOutMin=[]  SumDenOutMax=[]  SumNumOutMin=[]  SumNumOutMax=[]  DivideOutMin=[]  DivideOutMax=[]  UdiffTsProdOutMin=[]  UdiffTsProdOutMax=[]  NTsProdOutMin=[]  NTsProdOutMax=[]  UintegralTsProdOutMin=[]  UintegralTsProdOutMax=[]  UngainTsProdOutMin=[]  UngainTsProdOutMax=[]  ClampingZeroOutDataTypeStr=Inherit: Inherit via back propagation  ClampingZeroOutMin=[]  ClampingZeroOutMax=[]  FilterDenConstantOutDataTypeStr=Inherit: Inherit via back propagation  FilterDenConstantOutMin=[]  FilterDenConstantOutMax=[]  PCopyOutDataTypeStr=Inherit: Inherit via back propagation  PCopyOutMin=[]  PCopyOutMax=[]  NCopyOutDataTypeStr=Inherit: Inherit via back propagation  NCopyOutMin=[]  NCopyOutMax=[]  IntegratorContinuousStateAttributes=''  IntegratorStateMustResolveToSignalObject=off  IntegratorRTWStateStorageClass=Auto  FilterContinuousStateAttributes=''  FilterStateMustResolveToSignalObject=off  FilterRTWStateStorageClass=Auto  ParallelPVariant=InternalParameters  IdealPVariant=Disabled  IVariant=InternalParameters  DVariant=InternalParameters  IntegratorVariant=Continuous  SatVariant=Disabled  AWVariant=Passthrough  PCopyVariant=Disabled  TRVariant=Disabled  FdbkBlocksVariant=Forward  IdealPFdbkVariant=Disabled  SatFdbkVariant=Disabled  DerivativeFilterVariant=ContFilter  NVariant=InternalParameters  NCopyVariant=Disabled  FilterICVariant=InternalICsFilter  IntegratorICVariant=InternalICs  ExternalResetVariant=Disabled  TRSumVariant=Passthrough  SumFdbkVariant=Disabled  SumVariant=Sum_PID  TsampFilterVariant=InternalTs  TsampNgainVariant=Passthrough  TsampIntegralVariant=Passthrough  ExternalSaturationOutDataTypeStr=Inherit: Same as second input
  Saturation{,5..7} (4 alike) : Saturate  UpperLimit=50  LowerLimit=-50
  Saturation{1..4} (4 alike) : Saturate  UpperLimit=50  LowerLimit=0
  Scope : Scope  NumInputPorts=4
  Scope{1..4} (4 alike) : Scope  NumInputPorts=2
  Sum{,1..3,5..8} (8 alike) : Sum  Inputs=-+|
  Out1 : Outport
  wires:
  In1/1 -> Demux/1
  Demux/1 -> Sum/2
  Sum/1 -> PID Controller5/1
  Constant/1 -> Sum/1
  PID Controller5/1 -> Saturation/1
  Mux/1 -> Out1/1
  Saturation/1 -> Mux/1
  Saturation1/1 -> Scope/1, Mux/5
  Sum3/1 -> PID Controller1/1
  PID Controller1/1 -> Saturation1/1
  Demux/5 -> Sum3/2
  Constant1/1 -> Sum3/1
  Demux/8 -> Sum8/2, Scope1/2
  PID Controller4/1 -> Scope3/1, Saturation2/1
  Saturation2/1 -> Scope3/2, Scope/4, Mux/8
  Constant2/1 -> Sum8/1
  Demux/7 -> Sum1/2, Scope2/1
  Constant3/1 -> Sum1/1
  PID Controller3/1 -> Scope4/1, Saturation3/1
  Saturation3/1 -> Scope4/2, Scope/3, Mux/7
  Sum1/1 -> PID Controller3/1, Scope2/2
  Demux/6 -> Sum2/2
  Constant4/1 -> Sum2/1
  PID Controller2/1 -> Saturation4/1
  Saturation4/1 -> Scope/2, Mux/6
  Sum2/1 -> PID Controller2/1
  PID Controller6/1 -> Saturation5/1
  Constant5/1 -> Sum5/1
  Demux/2 -> Sum5/2
  Sum5/1 -> PID Controller6/1
  PID Controller7/1 -> Saturation6/1
  Constant6/1 -> Sum6/1
  Saturation6/1 -> Mux/3
  Demux/3 -> Sum6/2
  Sum6/1 -> PID Controller7/1
  Sum7/1 -> PID Controller8/1
  PID Controller8/1 -> Saturation7/1
  Demux/4 -> Sum7/2
  Constant7/1 -> Sum7/1
  Saturation7/1 -> Mux/4
  Saturation5/1 -> Mux/2
  Sum8/1 -> PID Controller4/1, Scope1/1

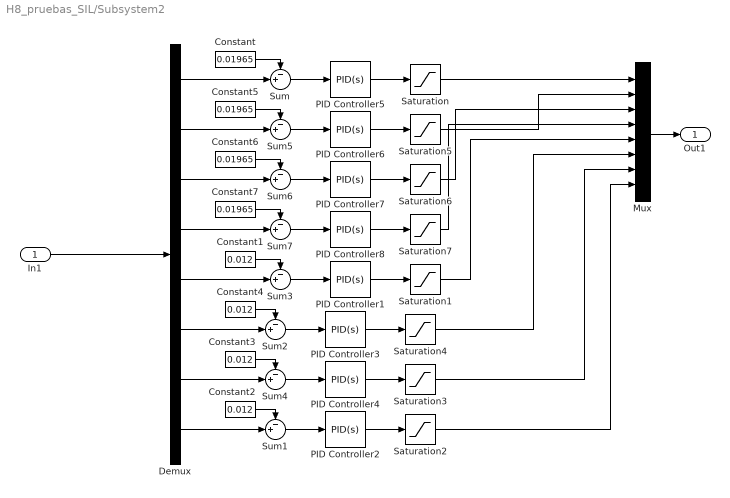
== system H8_pruebas_SIL/Subsystem2 ==
  In1 : Inport
  Constant{,5..7} (4 alike) : Constant  Value=0.01965
  Constant{1..4} (4 alike) : Constant  Value=0.012
  Demux : Demux  Outputs=8
  Mux : Mux  Inputs=8
  PID Controller{1..4} (4 alike) : slpidlib/PID Controller  Controller=PID  Form=Parallel  TimeDomain=Continuous-time  UseExternalTs=off  SampleTime=-1  IntegratorMethod=Forward Euler  FilterMethod=Forward Euler  ControllerParametersSource=internal  P=5490  I=10500  UseKiTs=off  D=350  N=1900  UseFilter=on  TunerSelectOption=Transfer Function Based (PID Tuner App)  InitialConditionSource=internal  InitialConditionForIntegrator=suelo  InitialConditionForFilter=0  DifferentiatorICPrevScaledInput=0  ExternalReset=none  TrackingMode=off  Kt=1  LimitOutput=off  SatLimitsSource=internal  UpperSaturationLimit=inf  LowerSaturationLimit=-inf  LinearizeAsGain=on  AntiWindupMode=none  Kb=1  LimitIntegrator=off  UpperIntegratorSaturationLimit=inf  LowerIntegratorSaturationLimit=-inf  POutMin=[]  POutMax=[]  IOutMin=[]  IOutMax=[]  DOutMin=[]  DOutMax=[]  NOutMin=[]  NOutMax=[]  SumOutMin=[]  SumOutMax=[]  SaturationOutMin=[]  SaturationOutMax=[]  PParamMin=[]  PParamMax=[]  IParamMin=[]  IParamMax=[]  DParamMin=[]  DParamMax=[]  NParamMin=[]  NParamMax=[]  KbParamMin=[]  KbParamMax=[]  KtParamMin=[]  KtParamMax=[]  KbOutMin=[]  KbOutMax=[]  KtOutMin=[]  KtOutMax=[]  IntegratorOutMin=[]  IntegratorOutMax=[]  FilterOutMin=[]  FilterOutMax=[]  SumI1OutMin=[]  SumI1OutMax=[]  SumI2OutMin=[]  SumI2OutMax=[]  SumI3OutMin=[]  SumI3OutMax=[]  SumI4OutMin=[]  SumI4OutMax=[]  SumDOutMin=[]  SumDOutMax=[]  DifferentiatorOutMin=[]  DifferentiatorOutMax=[]  FilterDiffOutCoefMin=[]  FilterDiffOutCoefMax=[]  ReciprocalOutMin=[]  ReciprocalOutMax=[]  SumDenOutMin=[]  SumDenOutMax=[]  SumNumOutMin=[]  SumNumOutMax=[]  DivideOutMin=[]  DivideOutMax=[]  UdiffTsProdOutMin=[]  UdiffTsProdOutMax=[]  NTsProdOutMin=[]  NTsProdOutMax=[]  UintegralTsProdOutMin=[]  UintegralTsProdOutMax=[]  UngainTsProdOutMin=[]  UngainTsProdOutMax=[]  ClampingZeroOutDataTypeStr=Inherit: Inherit via back propagation  ClampingZeroOutMin=[]  ClampingZeroOutMax=[]  FilterDenConstantOutDataTypeStr=Inherit: Inherit via back propagation  FilterDenConstantOutMin=[]  FilterDenConstantOutMax=[]  PCopyOutDataTypeStr=Inherit: Inherit via back propagation  PCopyOutMin=[]  PCopyOutMax=[]  NCopyOutDataTypeStr=Inherit: Inherit via back propagation  NCopyOutMin=[]  NCopyOutMax=[]  IntegratorContinuousStateAttributes=''  IntegratorStateMustResolveToSignalObject=off  IntegratorRTWStateStorageClass=Auto  FilterContinuousStateAttributes=''  FilterStateMustResolveToSignalObject=off  FilterRTWStateStorageClass=Auto  ParallelPVariant=InternalParameters  IdealPVariant=Disabled  IVariant=InternalParameters  DVariant=InternalParameters  IntegratorVariant=Continuous  SatVariant=Disabled  AWVariant=Passthrough  PCopyVariant=Disabled  TRVariant=Disabled  FdbkBlocksVariant=Forward  IdealPFdbkVariant=Disabled  SatFdbkVariant=Disabled  DerivativeFilterVariant=ContFilter  NVariant=InternalParameters  NCopyVariant=Disabled  FilterICVariant=InternalICsFilter  IntegratorICVariant=InternalICs  ExternalResetVariant=Disabled  TRSumVariant=Passthrough  SumFdbkVariant=Disabled  SumVariant=Sum_PID  TsampFilterVariant=InternalTs  TsampNgainVariant=Passthrough  TsampIntegralVariant=Passthrough  ExternalSaturationOutDataTypeStr=Inherit: Same as second input
  PID Controller{5..8} (4 alike) : slpidlib/PID Controller  Controller=PID  Form=Parallel  TimeDomain=Continuous-time  UseExternalTs=off  SampleTime=-1  IntegratorMethod=Forward Euler  FilterMethod=Forward Euler  ControllerParametersSource=internal  P=64900  I=155000  UseKiTs=off  D=1000  N=1900  UseFilter=on  TunerSelectOption=Transfer Function Based (PID Tuner App)  InitialConditionSource=internal  InitialConditionForIntegrator=suelo  InitialConditionForFilter=0  DifferentiatorICPrevScaledInput=0  ExternalReset=none  TrackingMode=off  Kt=1  LimitOutput=off  SatLimitsSource=internal  UpperSaturationLimit=inf  LowerSaturationLimit=-inf  LinearizeAsGain=on  AntiWindupMode=none  Kb=1  LimitIntegrator=off  UpperIntegratorSaturationLimit=inf  LowerIntegratorSaturationLimit=-inf  POutMin=[]  POutMax=[]  IOutMin=[]  IOutMax=[]  DOutMin=[]  DOutMax=[]  NOutMin=[]  NOutMax=[]  SumOutMin=[]  SumOutMax=[]  SaturationOutMin=[]  SaturationOutMax=[]  PParamMin=[]  PParamMax=[]  IParamMin=[]  IParamMax=[]  DParamMin=[]  DParamMax=[]  NParamMin=[]  NParamMax=[]  KbParamMin=[]  KbParamMax=[]  KtParamMin=[]  KtParamMax=[]  KbOutMin=[]  KbOutMax=[]  KtOutMin=[]  KtOutMax=[]  IntegratorOutMin=[]  IntegratorOutMax=[]  FilterOutMin=[]  FilterOutMax=[]  SumI1OutMin=[]  SumI1OutMax=[]  SumI2OutMin=[]  SumI2OutMax=[]  SumI3OutMin=[]  SumI3OutMax=[]  SumI4OutMin=[]  SumI4OutMax=[]  SumDOutMin=[]  SumDOutMax=[]  DifferentiatorOutMin=[]  DifferentiatorOutMax=[]  FilterDiffOutCoefMin=[]  FilterDiffOutCoefMax=[]  ReciprocalOutMin=[]  ReciprocalOutMax=[]  SumDenOutMin=[]  SumDenOutMax=[]  SumNumOutMin=[]  SumNumOutMax=[]  DivideOutMin=[]  DivideOutMax=[]  UdiffTsProdOutMin=[]  UdiffTsProdOutMax=[]  NTsProdOutMin=[]  NTsProdOutMax=[]  UintegralTsProdOutMin=[]  UintegralTsProdOutMax=[]  UngainTsProdOutMin=[]  UngainTsProdOutMax=[]  ClampingZeroOutDataTypeStr=Inherit: Inherit via back propagation  ClampingZeroOutMin=[]  ClampingZeroOutMax=[]  FilterDenConstantOutDataTypeStr=Inherit: Inherit via back propagation  FilterDenConstantOutMin=[]  FilterDenConstantOutMax=[]  PCopyOutDataTypeStr=Inherit: Inherit via back propagation  PCopyOutMin=[]  PCopyOutMax=[]  NCopyOutDataTypeStr=Inherit: Inherit via back propagation  NCopyOutMin=[]  NCopyOutMax=[]  IntegratorContinuousStateAttributes=''  IntegratorStateMustResolveToSignalObject=off  IntegratorRTWStateStorageClass=Auto  FilterContinuousStateAttributes=''  FilterStateMustResolveToSignalObject=off  FilterRTWStateStorageClass=Auto  ParallelPVariant=InternalParameters  IdealPVariant=Disabled  IVariant=InternalParameters  DVariant=InternalParameters  IntegratorVariant=Continuous  SatVariant=Disabled  AWVariant=Passthrough  PCopyVariant=Disabled  TRVariant=Disabled  FdbkBlocksVariant=Forward  IdealPFdbkVariant=Disabled  SatFdbkVariant=Disabled  DerivativeFilterVariant=ContFilter  NVariant=InternalParameters  NCopyVariant=Disabled  FilterICVariant=InternalICsFilter  IntegratorICVariant=InternalICs  ExternalResetVariant=Disabled  TRSumVariant=Passthrough  SumFdbkVariant=Disabled  SumVariant=Sum_PID  TsampFilterVariant=InternalTs  TsampNgainVariant=Passthrough  TsampIntegralVariant=Passthrough  ExternalSaturationOutDataTypeStr=Inherit: Same as second input
  Saturation{,5..7} (4 alike) : Saturate  UpperLimit=50  LowerLimit=-50
  Saturation{1..4} (4 alike) : Saturate  UpperLimit=50  LowerLimit=0
  Sum{,1..7} (8 alike) : Sum  Inputs=-+|
  Out1 : Outport
  wires:
  In1/1 -> Demux/1
  Demux/1 -> Sum/2
  Sum/1 -> PID Controller5/1
  Constant/1 -> Sum/1
  PID Controller5/1 -> Saturation/1
  Mux/1 -> Out1/1
  Saturation/1 -> Mux/1
  Saturation1/1 -> Mux/5
  Sum3/1 -> PID Controller1/1
  PID Controller1/1 -> Saturation1/1
  Demux/5 -> Sum3/2
  Constant1/1 -> Sum3/1
  Demux/6 -> Sum2/2
  Constant4/1 -> Sum2/1
  PID Controller3/1 -> Saturation4/1
  Saturation4/1 -> Mux/6
  Sum2/1 -> PID Controller3/1
  PID Controller6/1 -> Saturation5/1
  Constant5/1 -> Sum5/1
  Demux/2 -> Sum5/2
  Sum5/1 -> PID Controller6/1
  PID Controller7/1 -> Saturation6/1
  Constant6/1 -> Sum6/1
  Saturation6/1 -> Mux/3
  Demux/3 -> Sum6/2
  Sum6/1 -> PID Controller7/1
  Sum7/1 -> PID Controller8/1
  PID Controller8/1 -> Saturation7/1
  Demux/4 -> Sum7/2
  Constant7/1 -> Sum7/1
  Saturation7/1 -> Mux/4
  Saturation5/1 -> Mux/2
  Sum1/1 -> PID Controller2/1
  Demux/8 -> Sum1/2
  PID Controller2/1 -> Saturation2/1
  Constant2/1 -> Sum1/1
  Sum4/1 -> PID Controller4/1
  Demux/7 -> Sum4/2
  PID Controller4/1 -> Saturation3/1
  Constant3/1 -> Sum4/1
  Saturation3/1 -> Mux/7
  Saturation2/1 -> Mux/8

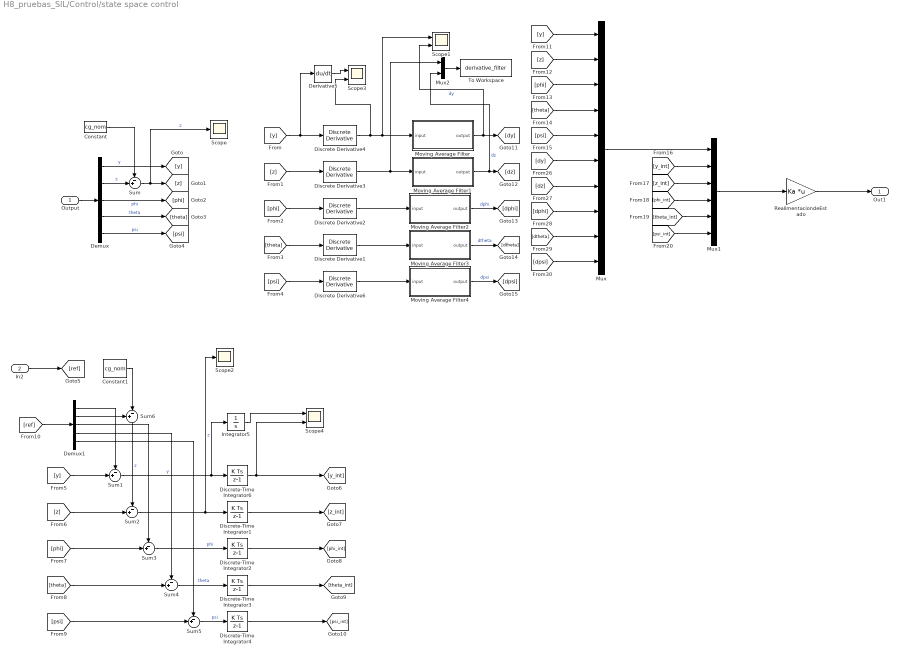
== system H8_pruebas_SIL/Control/state space control ==
  Output : Inport
  In2 : Inport  Port=2
  Constant : Constant  Value=cg_nom
  Constant1 : Constant  Value=cg_nom
  Demux : Demux  Outputs=5
  Demux1 : Demux  Outputs=5
  Derivative5 : Derivative
  Discrete Derivative{1..4,6} (5 alike) : simulink/Discrete/Discrete Derivative  gainval=1.0  ICPrevScaledInput=0.0  OutMin=[]  OutMax=[]  OutDataType=fixdt(1, 16)  OutScaling=2^-10  DoSatur=off
  Discrete-Time Integrator{1..4,6} (5 alike) : DiscreteIntegrator  SampleTime=0.001  ICPrevOutput=DiscIntNeverNeededParam  ICPrevScaledInput=DiscIntNeverNeededParam
  Integrator5 : Integrator
  Moving Average Filter : Subsystem  mask{M=20, fs=-1}
      mask prompts: M "Orden del filtro (M)"; fs "Frecuencia de muestreo (fs)"
  Moving Average Filter1 : Subsystem  mask{M=20, fs=-1}
      mask prompts: M "Orden del filtro (M)"; fs "Frecuencia de muestreo (fs)"
  Moving Average Filter2 : Subsystem  mask{M=20, fs=-1}
      mask prompts: M "Orden del filtro (M)"; fs "Frecuencia de muestreo (fs)"
  Moving Average Filter3 : Subsystem  mask{M=20, fs=-1}
      mask prompts: M "Orden del filtro (M)"; fs "Frecuencia de muestreo (fs)"
  Moving Average Filter4 : Subsystem  mask{M=20, fs=-1}
      mask prompts: M "Orden del filtro (M)"; fs "Frecuencia de muestreo (fs)"
  Mux : Mux  Inputs=10
  Mux1 : Mux  Inputs=6
  Mux2 : Mux  Inputs=2
  RealimentaciondeEstado : Gain  Gain=Ka  Multiplication=Matrix(K*u)
  Scope : Scope
  Scope1 : Scope  NumInputPorts=2
  Scope2 : Scope
  Scope3 : Scope  NumInputPorts=2
  Scope4 : Scope  NumInputPorts=2
  Sum{,1..5} (6 alike) : Sum  Inputs=-+|
  Sum6 : Sum  Inputs=+-|
  To Workspace : ToWorkspace  VariableName=derivative_filter  SaveFormat=Timeseries  SampleTime=-1
  Out1 : Outport
  wires:
  Output/1 -> Demux/1
  Discrete Derivative4/1 -> Scope3/2, Scope1/1, Moving Average Filter/1(input)
  Discrete Derivative3/1 -> Mux2/1, Moving Average Filter1/1(input)
  Discrete Derivative2/1 -> Moving Average Filter2/1(input)
  Discrete Derivative1/1 -> Moving Average Filter3/1(input)
  Discrete Derivative6/1 -> Moving Average Filter4/1(input)
  Mux/1 -> Mux1/1
  Demux/1 -> [y]  "y"
  Constant/1 -> Sum/1
  Sum/1 -> Scope/1, [z]  "z"
  Demux/2 -> Sum/2  "z"
  Demux/3 -> [phi]  "phi"
  Demux/4 -> [theta]  "theta"
  Demux/5 -> [psi]  "psi"
  [psi] -> Discrete Derivative6/1
  [theta] -> Discrete Derivative1/1
  [phi] -> Discrete Derivative2/1
  [z] -> Discrete Derivative3/1
  [y] -> Discrete Derivative4/1, Derivative5/1
  In2/1 -> [ref]
  [ref] -> Demux1/1
  [y] -> Sum1/2
  [z] -> Sum2/2
  [phi] -> Sum3/2
  [theta] -> Sum4/2
  [psi] -> Sum5/2
  Demux1/1 -> Sum1/1
  Demux1/3 -> Sum3/1
  Demux1/4 -> Sum4/1
  Demux1/5 -> Sum5/1
  Sum1/1 -> Discrete-Time Integrator6/1, Integrator5/1  "y"
  Sum5/1 -> Discrete-Time Integrator4/1  "psi"
  Sum4/1 -> Discrete-Time Integrator3/1  "theta"
  Sum3/1 -> Discrete-Time Integrator2/1  "phi"
  Sum2/1 -> Discrete-Time Integrator1/1, Scope2/1  "z"
  [y] -> Mux/1
  [z] -> Mux/2
  [phi] -> Mux/3
  [theta] -> Mux/4
  [psi] -> Mux/5
  Discrete-Time Integrator6/1 -> Scope4/2, [y_int]
  Discrete-Time Integrator1/1 -> [z_int]
  Discrete-Time Integrator2/1 -> [phi_int]
  Discrete-Time Integrator3/1 -> [theta_int]
  Moving Average Filter/1(output) -> [dy], Scope1/2  "dy"
  Moving Average Filter1/1(output) -> Mux2/2, [dz]  "dz"
  Moving Average Filter2/1(output) -> [dphi]  "dphi"
  Moving Average Filter4/1(output) -> [dpsi]  "dpsi"
  Moving Average Filter3/1(output) -> [dtheta]  "dtheta"
  [y_int] -> Mux1/2
  [psi_int] -> Mux1/6
  [theta_int] -> Mux1/5
  [phi_int] -> Mux1/4
  [z_int] -> Mux1/3
  Mux1/1 -> RealimentaciondeEstado/1
  Constant1/1 -> Sum6/2
  Demux1/2 -> Sum6/1
  Sum6/1 -> Sum2/1  "z"
  Discrete-Time Integrator4/1 -> [psi_int]
  [dtheta] -> Mux/9
  [dy] -> Mux/6
  [dz] -> Mux/7
  [dpsi] -> Mux/10
  [dphi] -> Mux/8
  RealimentaciondeEstado/1 -> Out1/1
  Mux2/1 -> To Workspace/1
  Integrator5/1 -> Scope4/1
  Derivative5/1 -> Scope3/1
